simulink model "SF016A_VehSpdLimr"  (R2013b)
settings: Solver=FixedStepDiscrete  StartTime=0.0  StopTime=15  FixedStep=.002  RelTol=1e-3
values from neighbouring files (symbols this model uses):
  VehSpdLimrMaxAssiY = DataDict.Calibration    [SF016A_VehSpdLimr_DataDict.m]
  VehSpdLimrPosMaxOffs1 = DataDict.Calibration    [SF016A_VehSpdLimr_DataDict.m]
  VehSpdLimrPosMaxOffs2 = DataDict.Calibration    [SF016A_VehSpdLimr_DataDict.m]
libraries: FloatToFixd x4, NxtrAbslt x3, simulink x1, FixdToFloat x1, NxtrLim x1, LnrIntrpnDyn x1, LnrIntrpn x1
settings Model: CovHTMLOptions=-aTS=1 -bRG=1 -bTC=1 -hTR=0 -nFC=0 -scm=1 -bcm=1 -xEv=0  Creator=Praveen/Muragesh (KPIT)  LastModifiedBy=BZHF94
settings DataIOCC: SignalLoggingSaveFormat=ModelDataLogs  SaveOutput=off  SignalLogging=off  DSMLogging=off  SaveTime=off
settings OptimizationCC: ExpressionDepthLimit=2147483647
settings DebuggingCC: SolverPrmCheckMsg=none  ParameterPrecisionLossMsg=none  FcnCallInpInsideContextMsg=UseLocalSettings  StateNameClashWarn=warning
settings GRTTargetCC: CombineOutputUpdateFcns=off  GRTInterface=on

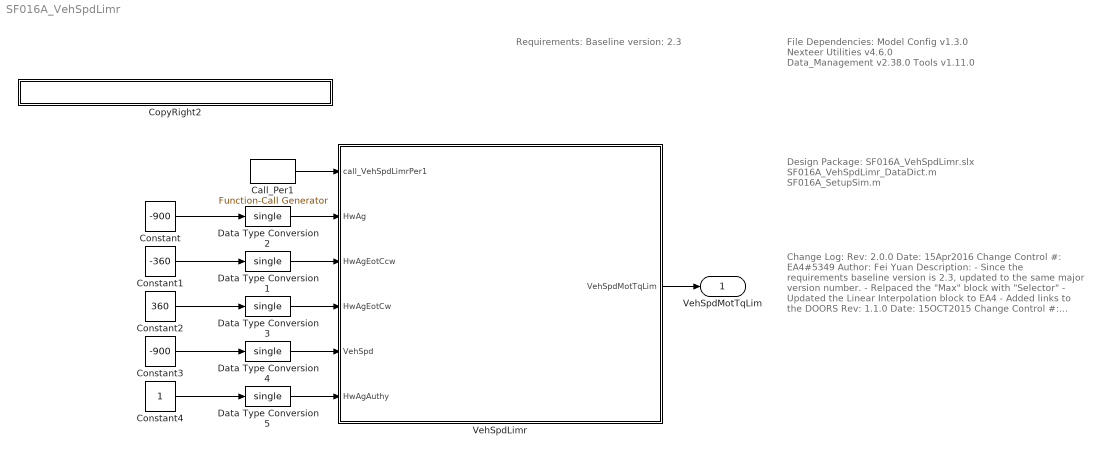
== system SF016A_VehSpdLimr ==
  note: File Dependencies:
      |
      | Model Config v1.3.0
      | Nexteer Utilities v4.6.0
      | Data_Management v2.38.0
      | Tools v1.11.0
  note: Requirements: Baseline version: 2.3
  note: Change Log:
      |
      | Rev: 2.0.0
      | Date: 15Apr2016
      | Change Control #: EA4#5349
      | Author: Fei Yuan
      | Description:
      | - Since the requirements baseline version
      |   is 2.3, updated to the same major version
      |   number.
      | - Relpaced the "Max" block with "Selector"
      | - Updated the Linear Interpolation block to
      |   EA4
      | - Added links to the DOORS
      |
      | Rev: 1.1.0
      | Date: 15OCT2015
      | Change Control #: EA4#1862
      | DRW: Praveen/Muragesh (KPIT)
      | Description:
      | Updated as per anomaly CR EA4#1276
      |
      |
      | Rev: 1.0.0
      | Date: 05AUG2015
      | Change Control #: EA4#513
      | DRW: Wheatley
      | Description:
      | Initial EA4 Release
      |  based on version EA3 v2.0
      |  this is a level 0 model
  note: Design Package:
      | SF016A_VehSpdLimr.slx
      | SF016A_VehSpdLimr_DataDict.m
      | SF016A_SetupSim.m
  Call_Per1 : simulink/Ports & Subsystems/Function-Call Generator  RequirementInfo="{'linktype_rmi_doors' '0000a52f (/E-STEER Core/SubSystem Specifications/Application Functions/SF016A Vehicle Speed Limiting)' '#SF016A_67' 'true' 'REQ:  SF016A_67' '' } %GIDa_4658042f_68a9_4f55_bcbd_8e644fae8943"  sample_time=0.002  numberOfIterations=1
  Constant : Constant  Value=-900
  Constant1 : Constant  Value=-360
  Constant2 : Constant  Value=360
  Constant3 : Constant  Value=-900
  Constant4 : Constant
  CopyRight2 : Subsystem  Description=|  mask(Copyright Information){none=on}
      | Copyright info block.                                               
      |                                                                     
      | Place copyright information at the top of every subsystem in design.
      mask prompts: none "No parameters"
      mask help: Place copyright information at the top of every subsystem in design.
      mask Display:
      | NxtrConf = 'Nexteer Confidential';
      | 
      | sys = bdroot; %handle for the current model ("system")
      | first = get_param(sys,'Created');
      | first = first(end-3:end);  %year is last four digits
      | 
      | last = get_param(sys,'LastModifiedDate');
      | if isempty(last)
      |     last = datestr(now,'yyyy');
      | else
      |     last = last(end-3:end);
      | end
      | 
      | if strcmp(first,last)
      |     fprintf('%s -- Copyright %s Nexteer',NxtrConf,first)
      | else
      |     fprintf('%s -- %s%s- %s Nexteer',NxtrConf,char(169),first,last)
      | end
  Data Type Conversion{1..5} (5 alike) : DataTypeConversion  OutDataTypeStr=single
  VehSpdLimr : Subsystem
  VehSpdMotTqLim : Outport  RequirementInfo={} %GIDa_da28f505_4b6b_4750_bcec_084d0a7cec68
  wires:
  VehSpdLimr/1(VehSpdMotTqLim) -> VehSpdMotTqLim/1
  Call_Per1/1 -> VehSpdLimr/1(call_VehSpdLimrPer1)
  Constant/1 -> Data Type Conversion2/1
  Constant1/1 -> Data Type Conversion1/1
  Constant2/1 -> Data Type Conversion3/1
  Data Type Conversion1/1 -> VehSpdLimr/3(HwAgEotCcw)
  Data Type Conversion3/1 -> VehSpdLimr/4(HwAgEotCw)
  Data Type Conversion2/1 -> VehSpdLimr/2(HwAg)
  Constant3/1 -> Data Type Conversion4/1
  Constant4/1 -> Data Type Conversion5/1
  Data Type Conversion5/1 -> VehSpdLimr/6(HwAgAuthy)
  Data Type Conversion4/1 -> VehSpdLimr/5(VehSpd)

== system SF016A_VehSpdLimr/CopyRight2 ==

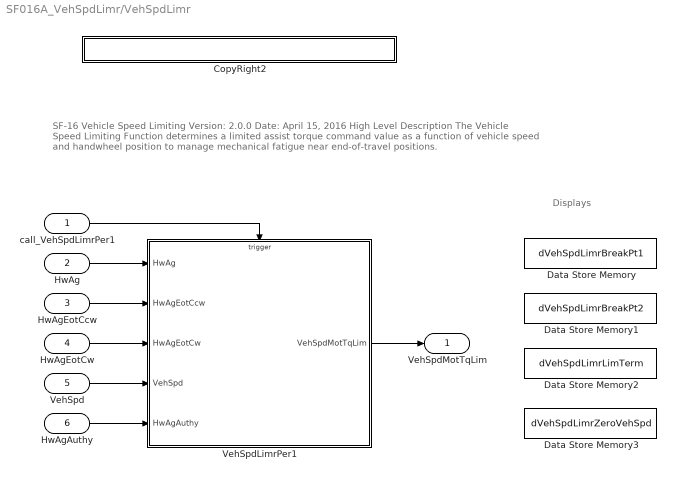
== system SF016A_VehSpdLimr/VehSpdLimr ==
  note: Displays
  note: SF-16  Vehicle Speed Limiting
      |          Version:  2.0.0                      Date:  April 15, 2016
      |
      |  High Level Description
      |      The Vehicle Speed Limiting Function determines a limited assist torque command value as a function of vehicle
      |      speed and handwheel position to manage mechanical fatigue near end-of-travel positions.
  call_VehSpdLimrPer1 : Inport
  HwAg : Inport  RequirementInfo="{'linktype_rmi_doors' '0000a52f (/E-STEER Core/SubSystem Specifications/Application Functions/SF016A Vehicle Speed Limiting)' '#SF016A_9' 'true' 'REQ:  SF016A_9' '' } %GIDa_20547f83_a8e8_4141_b0f2_e12d69f35c0f"  Port=2
  HwAgEotCcw : Inport  RequirementInfo="{'linktype_rmi_doors' '0000a52f (/E-STEER Core/SubSystem Specifications/Application Functions/SF016A Vehicle Speed Limiting)' '#SF016A_33' 'true' 'REQ:  SF016A_33' '' } %GIDa_3ac37e8a_9dbe_40a7_8cf1_05a3310f1eab"  Port=3
  HwAgEotCw : Inport  RequirementInfo="{'linktype_rmi_doors' '0000a52f (/E-STEER Core/SubSystem Specifications/Application Functions/SF016A Vehicle Speed Limiting)' '#SF016A_34' 'true' 'REQ:  SF016A_34' '' } %GIDa_e8ff42f4_7b63_425a_824a_61ddee63e2cb"  Port=4
  VehSpd : Inport  RequirementInfo="{'linktype_rmi_doors' '0000a52f (/E-STEER Core/SubSystem Specifications/Application Functions/SF016A Vehicle Speed Limiting)' '#SF016A_32' 'true' 'REQ:  SF016A_32' '' } %GIDa_d2851bec_d3f7_4000_a703_08ebed04af28"  Port=5
  HwAgAuthy : Inport  RequirementInfo="{'linktype_rmi_doors' '0000a52f (/E-STEER Core/SubSystem Specifications/Application Functions/SF016A Vehicle Speed Limiting)' '#SF016A_35' 'true' 'REQ:  SF016A_35' '' } %GIDa_755c219f_160e_44a1_8e53_1c7262d57e16"  Port=6
  CopyRight2 : Subsystem  Description=|  mask(Copyright Information){none=on}
      | Copyright info block.                                               
      |                                                                     
      | Place copyright information at the top of every subsystem in design.
      mask prompts: none "No parameters"
      mask help: Place copyright information at the top of every subsystem in design.
      mask Display:
      | NxtrConf = 'Nexteer Confidential';
      | 
      | sys = bdroot; %handle for the current model ("system")
      | first = get_param(sys,'Created');
      | first = first(end-3:end);  %year is last four digits
      | 
      | last = get_param(sys,'LastModifiedDate');
      | if isempty(last)
      |     last = datestr(now,'yyyy');
      | else
      |     last = last(end-3:end);
      | end
      | 
      | if strcmp(first,last)
      |     fprintf('%s -- Copyright %s Nexteer',NxtrConf,first)
      | else
      |     fprintf('%s -- %s%s- %s Nexteer',NxtrConf,char(169),first,last)
      | end
  Data Store Memory : DataStoreMemory  DataStoreName=dVehSpdLimrBreakPt1  ReadBeforeWriteMsg=warning  WriteAfterWriteMsg=warning  WriteAfterReadMsg=warning  StateMustResolveToSignalObject=on
  Data Store Memory1 : DataStoreMemory  DataStoreName=dVehSpdLimrBreakPt2  ReadBeforeWriteMsg=warning  WriteAfterWriteMsg=warning  WriteAfterReadMsg=warning  StateMustResolveToSignalObject=on
  Data Store Memory2 : DataStoreMemory  DataStoreName=dVehSpdLimrLimTerm  ReadBeforeWriteMsg=warning  WriteAfterWriteMsg=warning  WriteAfterReadMsg=warning  StateMustResolveToSignalObject=on
  Data Store Memory3 : DataStoreMemory  DataStoreName=dVehSpdLimrZeroVehSpd  ReadBeforeWriteMsg=warning  WriteAfterWriteMsg=warning  WriteAfterReadMsg=warning  StateMustResolveToSignalObject=on
  VehSpdLimrPer1 : Subsystem  RequirementInfo={} %GIDa_a7b0248b_b47a_44ce_9f08_25597632b35e
  VehSpdMotTqLim : Outport  RequirementInfo="{'linktype_rmi_doors' '0000a52f (/E-STEER Core/SubSystem Specifications/Application Functions/SF016A Vehicle Speed Limiting)' '#SF016A_71' 'true' 'REQ:  SF016A_71' '' } %GIDa_d0f1a28c_c8c7_42db_82c7_049fb0679538"
  wires:
  VehSpdLimrPer1/1(VehSpdMotTqLim) -> VehSpdMotTqLim/1
  HwAg/1 -> VehSpdLimrPer1/1(HwAg)
  HwAgEotCcw/1 -> VehSpdLimrPer1/2(HwAgEotCcw)
  HwAgEotCw/1 -> VehSpdLimrPer1/3(HwAgEotCw)
  call_VehSpdLimrPer1/1 -> VehSpdLimrPer1/Trigger
  VehSpd/1 -> VehSpdLimrPer1/4(VehSpd)
  HwAgAuthy/1 -> VehSpdLimrPer1/5(HwAgAuthy)

== system SF016A_VehSpdLimr/VehSpdLimr/CopyRight2 ==

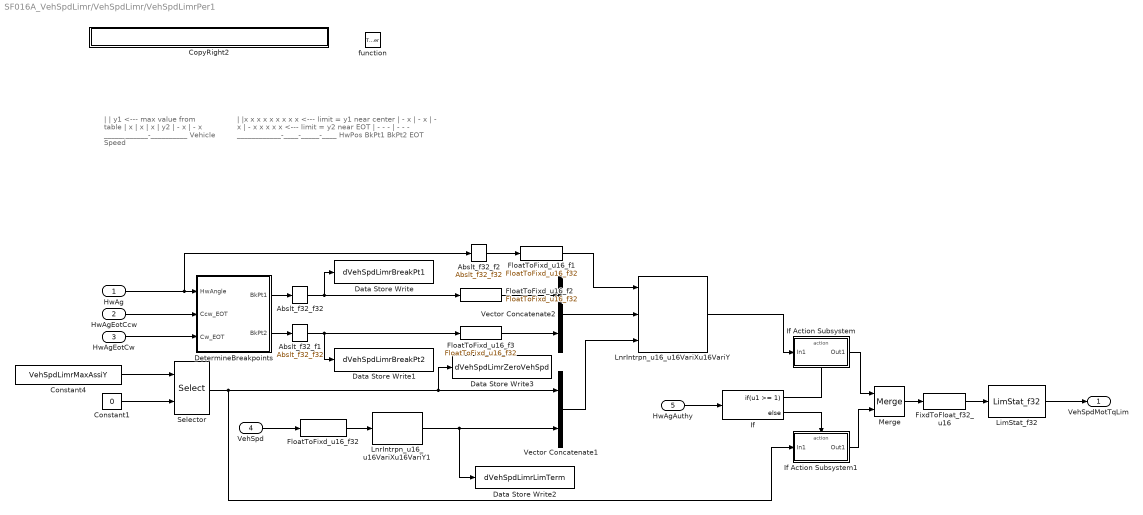
== system SF016A_VehSpdLimr/VehSpdLimr/VehSpdLimrPer1 ==
  note: |
      | | y1  <--- max value from table
      | |       x
      | |            x
      | |                 x
      | |                      y2
      | |                       -    x
      | |                       -         x
      | ____________-__________
      |               Vehicle Speed
  note: |
      | |x x x x x x x x x   <--- limit = y1 near center
      | |                       - x
      | |                       -   x
      | |                       -     x
      | |                       -        x x x x x   <--- limit = y2 near EOT
      | |                       -        -          -
      | |                       -        -          -
      | ____________-____-_____-____
      |  HwPos        BkPt1  BkPt2  EOT
  HwAg : Inport
  HwAgEotCcw : Inport  Port=2
  HwAgEotCw : Inport  Port=3
  VehSpd : Inport  Port=4
  HwAgAuthy : Inport  Port=5
  function : TriggerPort  TriggerType=function-call  PortDimensions=1
  Abslt_f32_f1 : NxtrAbslt/Abslt_f32_f32  RequirementInfo="{'linktype_rmi_doors' '0000a52f (/E-STEER Core/SubSystem Specifications/Application Functions/SF016A Vehicle Speed Limiting)' '#SF016A_56' 'true' 'REQ:  SF016A_56' '' ; 'linktype_rmi_doors' '0000a52f (/E-STEER Core/SubSystem Specifications/Application Functions/SF016A Vehicle Speed Limiting)' '#SF016A_54' 'true' 'REQ:  SF016A_54' '' } %GIDa_43263355_4d1a_4eb1_9e62_e416dfefd7d2"  SFunctionSpec=single y1 = Abslt_f32_f32(single u1)
      settings: AttributesFormatString=%<Name>
  Abslt_f32_f2 : NxtrAbslt/Abslt_f32_f32  RequirementInfo="{'linktype_rmi_doors' '0000a52f (/E-STEER Core/SubSystem Specifications/Application Functions/SF016A Vehicle Speed Limiting)' '#SF016A_56' 'true' 'REQ:  SF016A_56' '' } %GIDa_8eb8f50f_4865_40e8_a219_777cf0fc9352"  SFunctionSpec=single y1 = Abslt_f32_f32(single u1)
      settings: AttributesFormatString=%<Name>
  Abslt_f32_f32 : NxtrAbslt/Abslt_f32_f32  RequirementInfo="{'linktype_rmi_doors' '0000a52f (/E-STEER Core/SubSystem Specifications/Application Functions/SF016A Vehicle Speed Limiting)' '#SF016A_56' 'true' 'REQ:  SF016A_56' '' ; 'linktype_rmi_doors' '0000a52f (/E-STEER Core/SubSystem Specifications/Application Functions/SF016A Vehicle Speed Limiting)' '#SF016A_54' 'true' 'REQ:  SF016A_54' '' } %GIDa_6957cd74_7bb0_4d12_b411_ae19857dee05"  SFunctionSpec=single y1 = Abslt_f32_f32(single u1)
      settings: AttributesFormatString=%<Name>
  Constant1 : Constant  RequirementInfo={} %GIDa_2f2f3ffa_28ad_4d70_8ca4_c76dd9d21516  Value=0
  Constant4 : Constant  RequirementInfo="{'linktype_rmi_doors' '0000a52f (/E-STEER Core/SubSystem Specifications/Application Functions/SF016A Vehicle Speed Limiting)' '#SF016A_74' 'true' 'REQ:  SF016A_74' '' } %GIDa_3322659a_1957_4894_a58a_a65a58fad10f"  Value=VehSpdLimrMaxAssiY
  CopyRight2 : Subsystem  Description=|  mask(Copyright Information){none=on}
      | Copyright info block.                                               
      |                                                                     
      | Place copyright information at the top of every subsystem in design.
      mask prompts: none "No parameters"
      mask help: Place copyright information at the top of every subsystem in design.
      mask Display:
      | NxtrConf = 'Nexteer Confidential';
      | 
      | sys = bdroot; %handle for the current model ("system")
      | first = get_param(sys,'Created');
      | first = first(end-3:end);  %year is last four digits
      | 
      | last = get_param(sys,'LastModifiedDate');
      | if isempty(last)
      |     last = datestr(now,'yyyy');
      | else
      |     last = last(end-3:end);
      | end
      | 
      | if strcmp(first,last)
      |     fprintf('%s -- Copyright %s Nexteer',NxtrConf,first)
      | else
      |     fprintf('%s -- %s%s- %s Nexteer',NxtrConf,char(169),first,last)
      | end
  Data Store Write : DataStoreWrite  DataStoreName=dVehSpdLimrBreakPt1
  Data Store Write1 : DataStoreWrite  DataStoreName=dVehSpdLimrBreakPt2
  Data Store Write2 : DataStoreWrite  DataStoreName=dVehSpdLimrLimTerm
  Data Store Write3 : DataStoreWrite  DataStoreName=dVehSpdLimrZeroVehSpd
  DetermineBreakpoints : Subsystem  RequirementInfo="{'linktype_rmi_doors' '0000a52f (/E-STEER Core/SubSystem Specifications/Application Functions/SF016A Vehicle Speed Limiting)' '#SF016A_54' 'true' 'REQ:  SF016A_54' '' ; 'linktype_rmi_doors' '0000a52f (/E-STEER Core/SubSystem Specifications/Application Functions/SF016A Vehicle Speed Limiting)' '#SF016A_56' 'true' 'REQ:  SF016A_56' '' } %GIDa_640bd7c0_9db0_469b_8783_b292ad617612"
  FixdToFloat_f32_u16 : FixdToFloat/FixdToFloat_f32_u16  Param1=11
  FloatToFixd_u16_f1 : FloatToFixd/FloatToFixd_u16_f32  Param1=5
  FloatToFixd_u16_f2 : FloatToFixd/FloatToFixd_u16_f32  Param1=5
  FloatToFixd_u16_f3 : FloatToFixd/FloatToFixd_u16_f32  Param1=5
  FloatToFixd_u16_f32 : FloatToFixd/FloatToFixd_u16_f32  Param1=7
  If : If  RequirementInfo="{'linktype_rmi_doors' '0000a52f (/E-STEER Core/SubSystem Specifications/Application Functions/SF016A Vehicle Speed Limiting)' '#SF016A_75' 'true' 'REQ:  SF016A_75' '' ; 'linktype_rmi_doors' '0000a52f (/E-STEER Core/SubSystem Specifications/Application Functions/SF016A Vehicle Speed Limiting)' '#SF016A_54' 'true' 'REQ:  SF016A_54' '' ; 'linktype_rmi_doors' '0000a52f (/E-STEER Core/SubSystem Specifications/Application Functions/SF016A Vehicle Speed Limiting)' '#SF016A_58' 'true' 'REQ:  SF016A_58' '' ; 'linktype_rmi_doors' '0000a52f (/E-STEER Core/SubSystem Specifications/Application Functions/SF016A Vehicle Speed Limiting)' '#SF016A_59' 'true' 'REQ:  SF016A_59' '' } %GIDa_5033a59a_14fc_4531_96fc_5b75a1e94d2f"  IfExpression=u1 >= 1
  If Action Subsystem : Subsystem  RequirementInfo="{'linktype_rmi_doors' '0000a52f (/E-STEER Core/SubSystem Specifications/Application Functions/SF016A Vehicle Speed Limiting)' '#SF016A_54' 'true' 'REQ:  SF016A_54' '' ; 'linktype_rmi_doors' '0000a52f (/E-STEER Core/SubSystem Specifications/Application Functions/SF016A Vehicle Speed Limiting)' '#SF016A_58' 'true' 'REQ:  SF016A_58' '' ; 'linktype_rmi_doors' '0000a52f (/E-STEER Core/SubSystem Specifications/Application Functions/SF016A Vehicle Speed Limiting)' '#SF016A_59' 'true' 'REQ:  SF016A_59' '' } %GIDa_86a6a176_9baa_4b24_9f35_1d44feccd65f"  TreatAsAtomicUnit=on
  If Action Subsystem1 : Subsystem  RequirementInfo="{'linktype_rmi_doors' '0000a52f (/E-STEER Core/SubSystem Specifications/Application Functions/SF016A Vehicle Speed Limiting)' '#SF016A_75' 'true' 'REQ:  SF016A_75' '' ; 'linktype_rmi_doors' '0000a52f (/E-STEER Core/SubSystem Specifications/Application Functions/SF016A Vehicle Speed Limiting)' '#SF016A_58' 'true' 'REQ:  SF016A_58' '' ; 'linktype_rmi_doors' '0000a52f (/E-STEER Core/SubSystem Specifications/Application Functions/SF016A Vehicle Speed Limiting)' '#SF016A_59' 'true' 'REQ:  SF016A_59' '' } %GIDa_13070b2b_abb9_4f1f_8896_3ac05b76473f"  TreatAsAtomicUnit=on
  LimStat_f32 : NxtrLim/LimStat_f32  RequirementInfo="{'linktype_rmi_doors' '0000a52f (/E-STEER Core/SubSystem Specifications/Application Functions/SF016A Vehicle Speed Limiting)' '#SF016A_66' 'true' 'REQ:  SF016A_66' '' } %GIDa_b7f64418_05a1_4509_9d3e_29ff1aafe1ab"  LoLim=SYSGLBPRM_MOTTQCMDLOLIM_MOTNWTMTR_F32  HiLim=SYSGLBPRM_MOTTQCMDHILIM_MOTNWTMTR_F32
      settings: AttributesFormatString=|
      | Low Limit: %<LoLim>
      | High Limit:%<HiLim>
  LnrIntrpn_u16_u16VariXu16VariY : LnrIntrpnDyn/LnrIntrpn_u16_u16VariXu16VariY  RequirementInfo="{'linktype_rmi_doors' '0000a52f (/E-STEER Core/SubSystem Specifications/Application Functions/SF016A Vehicle Speed Limiting)' '#SF016A_54' 'true' 'REQ:  SF016A_54' '' ; 'linktype_rmi_doors' '0000a52f (/E-STEER Core/SubSystem Specifications/Application Functions/SF016A Vehicle Speed Limiting)' '#SF016A_56' 'true' 'REQ:  SF016A_56' '' ; 'linktype_rmi_doors' '0000a52f (/E-STEER Core/SubSystem Specifications/Application Functions/SF016A Vehicle Speed Limiting)' '#SF016A_58' 'true' 'REQ:  SF016A_58' '' ; 'linktype_rmi_doors' '0000a52f (/E-STEER Core/SubSystem Specifications/Application Functions/SF016A Vehicle Speed Limiting)' '#SF016A_59' 'true' 'REQ:  SF016A_59' '' } %GIDa_2a3c4297_300c_4538_93a7_e8369b10a31f"
      settings: AttributesFormatString=Lnr ( u16VariX , u16VariY )
  LnrIntrpn_u16_u16VariXu16VariY1 : LnrIntrpn/LnrIntrpn_u16_u16VariXu16VariY  RequirementInfo="{'linktype_rmi_doors' '0000a52f (/E-STEER Core/SubSystem Specifications/Application Functions/SF016A Vehicle Speed Limiting)' '#SF016A_58' 'true' 'REQ:  SF016A_58' '' ; 'linktype_rmi_doors' '0000a52f (/E-STEER Core/SubSystem Specifications/Application Functions/SF016A Vehicle Speed Limiting)' '#SF016A_59' 'true' 'REQ:  SF016A_59' '' ; 'linktype_rmi_doors' '0000a52f (/E-STEER Core/SubSystem Specifications/Application Functions/SF016A Vehicle Speed Limiting)' '#SF016A_63' 'true' 'REQ:  SF016A_63' '' } %GIDa_7e84c74c_bad8_4c0d_9f88_70828bbee0f2"  XTbl=VehSpdLimrMaxAssiX  YTbl=VehSpdLimrMaxAssiY
      settings: AttributesFormatString=Lnr ( u16VariX , u16VariY )
  Merge : Merge  RequirementInfo="{'linktype_rmi_doors' '0000a52f (/E-STEER Core/SubSystem Specifications/Application Functions/SF016A Vehicle Speed Limiting)' '#SF016A_75' 'true' 'REQ:  SF016A_75' '' ; 'linktype_rmi_doors' '0000a52f (/E-STEER Core/SubSystem Specifications/Application Functions/SF016A Vehicle Speed Limiting)' '#SF016A_54' 'true' 'REQ:  SF016A_54' '' ; 'linktype_rmi_doors' '0000a52f (/E-STEER Core/SubSystem Specifications/Application Functions/SF016A Vehicle Speed Limiting)' '#SF016A_58' 'true' 'REQ:  SF016A_58' '' ; 'linktype_rmi_doors' '0000a52f (/E-STEER Core/SubSystem Specifications/Application Functions/SF016A Vehicle Speed Limiting)' '#SF016A_59' 'true' 'REQ:  SF016A_59' '' } %GIDa_04d40666_89e5_49bf_be68_7e9bf64bae41"
  Selector : Selector  RequirementInfo="{'linktype_rmi_doors' '0000a52f (/E-STEER Core/SubSystem Specifications/Application Functions/SF016A Vehicle Speed Limiting)' '#SF016A_75' 'true' 'REQ:  SF016A_75' '' } %GIDa_ed021c59_1b39_418e_9ab3_afd0e64960ef"  IndexMode=Zero-based  InputPortWidth=5  IndexOptions=Index vector (port)  Indices=[1 3]  OutputSizes=1
  Vector Concatenate1 : Concatenate  RequirementInfo="{'linktype_rmi_doors' '0000a52f (/E-STEER Core/SubSystem Specifications/Application Functions/SF016A Vehicle Speed Limiting)' '#SF016A_54' 'true' 'REQ:  SF016A_54' '' ; 'linktype_rmi_doors' '0000a52f (/E-STEER Core/SubSystem Specifications/Application Functions/SF016A Vehicle Speed Limiting)' '#SF016A_56' 'true' 'REQ:  SF016A_56' '' ; 'linktype_rmi_doors' '0000a52f (/E-STEER Core/SubSystem Specifications/Application Functions/SF016A Vehicle Speed Limiting)' '#SF016A_58' 'true' 'REQ:  SF016A_58' '' ; 'linktype_rmi_doors' '0000a52f (/E-STEER Core/SubSystem Specifications/Application Functions/SF016A Vehicle Speed Limiting)' '#SF016A_59' 'true' 'REQ:  SF016A_59' '' } %GIDa_aa604e0a_c245_4d50_bf5a_9e569c9abc5e"
  Vector Concatenate2 : Concatenate  RequirementInfo="{'linktype_rmi_doors' '0000a52f (/E-STEER Core/SubSystem Specifications/Application Functions/SF016A Vehicle Speed Limiting)' '#SF016A_54' 'true' 'REQ:  SF016A_54' '' ; 'linktype_rmi_doors' '0000a52f (/E-STEER Core/SubSystem Specifications/Application Functions/SF016A Vehicle Speed Limiting)' '#SF016A_56' 'true' 'REQ:  SF016A_56' '' ; 'linktype_rmi_doors' '0000a52f (/E-STEER Core/SubSystem Specifications/Application Functions/SF016A Vehicle Speed Limiting)' '#SF016A_58' 'true' 'REQ:  SF016A_58' '' ; 'linktype_rmi_doors' '0000a52f (/E-STEER Core/SubSystem Specifications/Application Functions/SF016A Vehicle Speed Limiting)' '#SF016A_59' 'true' 'REQ:  SF016A_59' '' } %GIDa_62854488_0536_41b3_903d_0888355aa9ab"
  VehSpdMotTqLim : Outport
  wires:
  DetermineBreakpoints/1(BkPt1) -> Abslt_f32_f32/1
  DetermineBreakpoints/2(BkPt2) -> Abslt_f32_f1/1
  HwAgAuthy/1 -> If/1
  HwAgEotCcw/1 -> DetermineBreakpoints/2(Ccw_EOT)
  HwAgEotCw/1 -> DetermineBreakpoints/3(Cw_EOT)
  Abslt_f32_f2/1 -> FloatToFixd_u16_f1/1
  HwAg/1 -> Abslt_f32_f2/1, DetermineBreakpoints/1(HwAngle)
  If/1 -> If Action Subsystem/Action
  If/2 -> If Action Subsystem1/Action
  If Action Subsystem/1(Out1) -> Merge/1
  If Action Subsystem1/1(Out1) -> Merge/2
  Merge/1 -> FixdToFloat_f32_u16/1
  LnrIntrpn_u16_u16VariXu16VariY/1 -> If Action Subsystem/1(In1)
  LimStat_f32/1 -> VehSpdMotTqLim/1
  FixdToFloat_f32_u16/1 -> LimStat_f32/1
  Vector Concatenate2/1 -> LnrIntrpn_u16_u16VariXu16VariY/2
  FloatToFixd_u16_f1/1 -> LnrIntrpn_u16_u16VariXu16VariY/1
  FloatToFixd_u16_f2/1 -> Vector Concatenate2/1
  FloatToFixd_u16_f3/1 -> Vector Concatenate2/2
  VehSpd/1 -> FloatToFixd_u16_f32/1
  FloatToFixd_u16_f32/1 -> LnrIntrpn_u16_u16VariXu16VariY1/1
  LnrIntrpn_u16_u16VariXu16VariY1/1 -> Data Store Write2/1, Vector Concatenate1/2
  Abslt_f32_f32/1 -> Data Store Write/1, FloatToFixd_u16_f2/1
  Abslt_f32_f1/1 -> Data Store Write1/1, FloatToFixd_u16_f3/1
  Selector/1 -> If Action Subsystem1/1(In1), Vector Concatenate1/1, Data Store Write3/1
  Vector Concatenate1/1 -> LnrIntrpn_u16_u16VariXu16VariY/3
  Constant1/1 -> Selector/2
  Constant4/1 -> Selector/1

== system SF016A_VehSpdLimr/VehSpdLimr/VehSpdLimrPer1/CopyRight2 ==

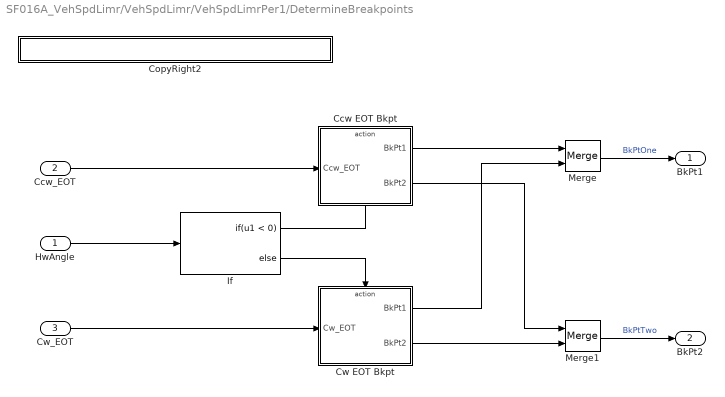
== system SF016A_VehSpdLimr/VehSpdLimr/VehSpdLimrPer1/DetermineBreakpoints ==
  HwAngle : Inport
  Ccw_EOT : Inport  Port=2
  Cw_EOT : Inport  Port=3
  Ccw EOT Bkpt : Subsystem  RequirementInfo="{'linktype_rmi_doors' '0000a52f (/E-STEER Core/SubSystem Specifications/Application Functions/SF016A Vehicle Speed Limiting)' '#SF016A_54' 'true' 'REQ:  SF016A_54' '' ; 'linktype_rmi_doors' '0000a52f (/E-STEER Core/SubSystem Specifications/Application Functions/SF016A Vehicle Speed Limiting)' '#SF016A_56' 'true' 'REQ:  SF016A_56' '' } %GIDa_e3c79417_19a6_48dc_9488_a36fc9b8a269"  TreatAsAtomicUnit=on
  CopyRight2 : Subsystem  Description=|  mask(Copyright Information){none=on}
      | Copyright info block.                                               
      |                                                                     
      | Place copyright information at the top of every subsystem in design.
      mask prompts: none "No parameters"
      mask help: Place copyright information at the top of every subsystem in design.
      mask Display:
      | NxtrConf = 'Nexteer Confidential';
      | 
      | sys = bdroot; %handle for the current model ("system")
      | first = get_param(sys,'Created');
      | first = first(end-3:end);  %year is last four digits
      | 
      | last = get_param(sys,'LastModifiedDate');
      | if isempty(last)
      |     last = datestr(now,'yyyy');
      | else
      |     last = last(end-3:end);
      | end
      | 
      | if strcmp(first,last)
      |     fprintf('%s -- Copyright %s Nexteer',NxtrConf,first)
      | else
      |     fprintf('%s -- %s%s- %s Nexteer',NxtrConf,char(169),first,last)
      | end
  Cw EOT Bkpt : Subsystem  RequirementInfo="{'linktype_rmi_doors' '0000a52f (/E-STEER Core/SubSystem Specifications/Application Functions/SF016A Vehicle Speed Limiting)' '#SF016A_54' 'true' 'REQ:  SF016A_54' '' ; 'linktype_rmi_doors' '0000a52f (/E-STEER Core/SubSystem Specifications/Application Functions/SF016A Vehicle Speed Limiting)' '#SF016A_56' 'true' 'REQ:  SF016A_56' '' } %GIDa_adf71e24_21ac_428d_a2e4_a099c634c138"  TreatAsAtomicUnit=on
  If : If  RequirementInfo="{'linktype_rmi_doors' '0000a52f (/E-STEER Core/SubSystem Specifications/Application Functions/SF016A Vehicle Speed Limiting)' '#SF016A_54' 'true' 'REQ:  SF016A_54' '' ; 'linktype_rmi_doors' '0000a52f (/E-STEER Core/SubSystem Specifications/Application Functions/SF016A Vehicle Speed Limiting)' '#SF016A_56' 'true' 'REQ:  SF016A_56' '' } %GIDa_c3b2335f_bbf3_490b_aa88_e7162cc8d21d"  IfExpression=u1 < 0
  Merge : Merge  RequirementInfo="{'linktype_rmi_doors' '0000a52f (/E-STEER Core/SubSystem Specifications/Application Functions/SF016A Vehicle Speed Limiting)' '#SF016A_54' 'true' 'REQ:  SF016A_54' '' ; 'linktype_rmi_doors' '0000a52f (/E-STEER Core/SubSystem Specifications/Application Functions/SF016A Vehicle Speed Limiting)' '#SF016A_56' 'true' 'REQ:  SF016A_56' '' } %GIDa_04a606ba_b5f0_43c7_bb3d_819425f6e791"
  Merge1 : Merge  RequirementInfo="{'linktype_rmi_doors' '0000a52f (/E-STEER Core/SubSystem Specifications/Application Functions/SF016A Vehicle Speed Limiting)' '#SF016A_54' 'true' 'REQ:  SF016A_54' '' ; 'linktype_rmi_doors' '0000a52f (/E-STEER Core/SubSystem Specifications/Application Functions/SF016A Vehicle Speed Limiting)' '#SF016A_56' 'true' 'REQ:  SF016A_56' '' } %GIDa_5b2318de_e3dc_4ba1_8390_700fb8f2154c"
  BkPt1 : Outport
  BkPt2 : Outport  Port=2
  wires:
  Ccw_EOT/1 -> Ccw EOT Bkpt/1(Ccw_EOT)
  Cw_EOT/1 -> Cw EOT Bkpt/1(Cw_EOT)
  If/1 -> Ccw EOT Bkpt/Action
  If/2 -> Cw EOT Bkpt/Action
  Ccw EOT Bkpt/1(BkPt1) -> Merge/1
  Cw EOT Bkpt/1(BkPt1) -> Merge/2
  Ccw EOT Bkpt/2(BkPt2) -> Merge1/1
  Cw EOT Bkpt/2(BkPt2) -> Merge1/2
  HwAngle/1 -> If/1
  Merge/1 -> BkPt1/1  "BkPtOne"
  Merge1/1 -> BkPt2/1  "BkPtTwo"

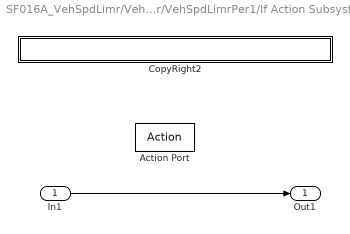
== system SF016A_VehSpdLimr/VehSpdLimr/VehSpdLimrPer1/If Action Subsystem ==
  In1 : Inport
  Action Port : ActionPort  ActionType=then
  CopyRight2 : Subsystem  Description=|  mask(Copyright Information){none=on}
      | Copyright info block.                                               
      |                                                                     
      | Place copyright information at the top of every subsystem in design.
      mask prompts: none "No parameters"
      mask help: Place copyright information at the top of every subsystem in design.
      mask Display:
      | NxtrConf = 'Nexteer Confidential';
      | 
      | sys = bdroot; %handle for the current model ("system")
      | first = get_param(sys,'Created');
      | first = first(end-3:end);  %year is last four digits
      | 
      | last = get_param(sys,'LastModifiedDate');
      | if isempty(last)
      |     last = datestr(now,'yyyy');
      | else
      |     last = last(end-3:end);
      | end
      | 
      | if strcmp(first,last)
      |     fprintf('%s -- Copyright %s Nexteer',NxtrConf,first)
      | else
      |     fprintf('%s -- %s%s- %s Nexteer',NxtrConf,char(169),first,last)
      | end
  Out1 : Outport
  wires:
  In1/1 -> Out1/1

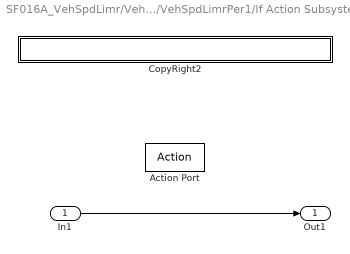
== system SF016A_VehSpdLimr/VehSpdLimr/VehSpdLimrPer1/If Action Subsystem1 ==
  In1 : Inport
  Action Port : ActionPort  ActionType=else
  CopyRight2 : Subsystem  Description=|  mask(Copyright Information){none=on}
      | Copyright info block.                                               
      |                                                                     
      | Place copyright information at the top of every subsystem in design.
      mask prompts: none "No parameters"
      mask help: Place copyright information at the top of every subsystem in design.
      mask Display:
      | NxtrConf = 'Nexteer Confidential';
      | 
      | sys = bdroot; %handle for the current model ("system")
      | first = get_param(sys,'Created');
      | first = first(end-3:end);  %year is last four digits
      | 
      | last = get_param(sys,'LastModifiedDate');
      | if isempty(last)
      |     last = datestr(now,'yyyy');
      | else
      |     last = last(end-3:end);
      | end
      | 
      | if strcmp(first,last)
      |     fprintf('%s -- Copyright %s Nexteer',NxtrConf,first)
      | else
      |     fprintf('%s -- %s%s- %s Nexteer',NxtrConf,char(169),first,last)
      | end
  Out1 : Outport
  wires:
  In1/1 -> Out1/1

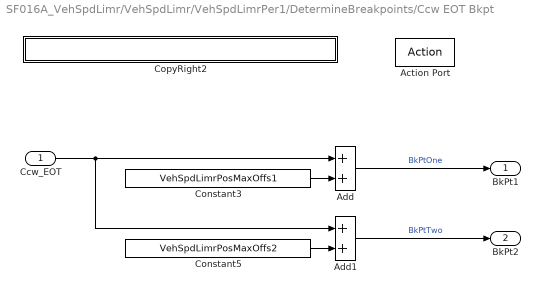
== system SF016A_VehSpdLimr/VehSpdLimr/VehSpdLimrPer1/DetermineBreakpoints/Ccw EOT Bkpt ==
  Ccw_EOT : Inport
  Action Port : ActionPort  ActionType=then
  Add : Sum  RequirementInfo="{'linktype_rmi_doors' '0000a52f (/E-STEER Core/SubSystem Specifications/Application Functions/SF016A Vehicle Speed Limiting)' '#SF016A_61' 'true' 'REQ:  SF016A_61' '' } %GIDa_b3801fec_f8e8_4979_97e6_a2343a16ea21"
  Add1 : Sum  RequirementInfo="{'linktype_rmi_doors' '0000a52f (/E-STEER Core/SubSystem Specifications/Application Functions/SF016A Vehicle Speed Limiting)' '#SF016A_62' 'true' 'REQ:  SF016A_62' '' } %GIDa_39bae563_2591_4b9f_ad28_0357182f1eb7"
  Constant3 : Constant  RequirementInfo="{'linktype_rmi_doors' '0000a52f (/E-STEER Core/SubSystem Specifications/Application Functions/SF016A Vehicle Speed Limiting)' '#SF016A_61' 'true' 'REQ:  SF016A_61' '' } %GIDa_66d15d56_bc81_42e3_bcd0_8a3b5ee1f4d3"  Value=VehSpdLimrPosMaxOffs1
  Constant5 : Constant  RequirementInfo="{'linktype_rmi_doors' '0000a52f (/E-STEER Core/SubSystem Specifications/Application Functions/SF016A Vehicle Speed Limiting)' '#SF016A_62' 'true' 'REQ:  SF016A_62' '' } %GIDa_c86c2d4f_1f1d_4609_ae27_bb0b7f5715ab"  Value=VehSpdLimrPosMaxOffs2
  CopyRight2 : Subsystem  Description=|  mask(Copyright Information){none=on}
      | Copyright info block.                                               
      |                                                                     
      | Place copyright information at the top of every subsystem in design.
      mask prompts: none "No parameters"
      mask help: Place copyright information at the top of every subsystem in design.
      mask Display:
      | NxtrConf = 'Nexteer Confidential';
      | 
      | sys = bdroot; %handle for the current model ("system")
      | first = get_param(sys,'Created');
      | first = first(end-3:end);  %year is last four digits
      | 
      | last = get_param(sys,'LastModifiedDate');
      | if isempty(last)
      |     last = datestr(now,'yyyy');
      | else
      |     last = last(end-3:end);
      | end
      | 
      | if strcmp(first,last)
      |     fprintf('%s -- Copyright %s Nexteer',NxtrConf,first)
      | else
      |     fprintf('%s -- %s%s- %s Nexteer',NxtrConf,char(169),first,last)
      | end
  BkPt1 : Outport
  BkPt2 : Outport  Port=2
  wires:
  Ccw_EOT/1 -> Add/1, Add1/1
  Constant3/1 -> Add/2
  Add/1 -> BkPt1/1  "BkPtOne"
  Constant5/1 -> Add1/2
  Add1/1 -> BkPt2/1  "BkPtTwo"

== system SF016A_VehSpdLimr/VehSpdLimr/VehSpdLimrPer1/DetermineBreakpoints/CopyRight2 ==

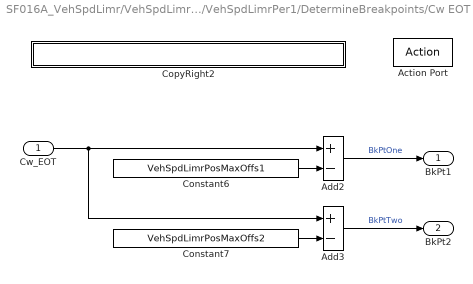
== system SF016A_VehSpdLimr/VehSpdLimr/VehSpdLimrPer1/DetermineBreakpoints/Cw EOT Bkpt ==
  Cw_EOT : Inport
  Action Port : ActionPort  ActionType=else
  Add2 : Sum  RequirementInfo="{'linktype_rmi_doors' '0000a52f (/E-STEER Core/SubSystem Specifications/Application Functions/SF016A Vehicle Speed Limiting)' '#SF016A_61' 'true' 'REQ:  SF016A_61' '' } %GIDa_8c079889_0248_4e08_800b_0d39e26c5b9e"  Inputs=+-
  Add3 : Sum  RequirementInfo="{'linktype_rmi_doors' '0000a52f (/E-STEER Core/SubSystem Specifications/Application Functions/SF016A Vehicle Speed Limiting)' '#SF016A_62' 'true' 'REQ:  SF016A_62' '' } %GIDa_5232dd6e_b17a_4e57_9522_b512f3e399d8"  Inputs=+-
  Constant6 : Constant  RequirementInfo="{'linktype_rmi_doors' '0000a52f (/E-STEER Core/SubSystem Specifications/Application Functions/SF016A Vehicle Speed Limiting)' '#SF016A_61' 'true' 'REQ:  SF016A_61' '' } %GIDa_8c3abd57_3412_4b35_b8e5_451f0f7225ed"  Value=VehSpdLimrPosMaxOffs1
  Constant7 : Constant  RequirementInfo="{'linktype_rmi_doors' '0000a52f (/E-STEER Core/SubSystem Specifications/Application Functions/SF016A Vehicle Speed Limiting)' '#SF016A_62' 'true' 'REQ:  SF016A_62' '' } %GIDa_f4fc982b_3fea_4ebf_bb74_65892309d805"  Value=VehSpdLimrPosMaxOffs2
  CopyRight2 : Subsystem  Description=|  mask(Copyright Information){none=on}
      | Copyright info block.                                               
      |                                                                     
      | Place copyright information at the top of every subsystem in design.
      mask prompts: none "No parameters"
      mask help: Place copyright information at the top of every subsystem in design.
      mask Display:
      | NxtrConf = 'Nexteer Confidential';
      | 
      | sys = bdroot; %handle for the current model ("system")
      | first = get_param(sys,'Created');
      | first = first(end-3:end);  %year is last four digits
      | 
      | last = get_param(sys,'LastModifiedDate');
      | if isempty(last)
      |     last = datestr(now,'yyyy');
      | else
      |     last = last(end-3:end);
      | end
      | 
      | if strcmp(first,last)
      |     fprintf('%s -- Copyright %s Nexteer',NxtrConf,first)
      | else
      |     fprintf('%s -- %s%s- %s Nexteer',NxtrConf,char(169),first,last)
      | end
  BkPt1 : Outport
  BkPt2 : Outport  Port=2
  wires:
  Cw_EOT/1 -> Add2/1, Add3/1
  Constant6/1 -> Add2/2
  Add2/1 -> BkPt1/1  "BkPtOne"
  Constant7/1 -> Add3/2
  Add3/1 -> BkPt2/1  "BkPtTwo"

== system SF016A_VehSpdLimr/VehSpdLimr/VehSpdLimrPer1/If Action Subsystem/CopyRight2 ==

== system SF016A_VehSpdLimr/VehSpdLimr/VehSpdLimrPer1/If Action Subsystem1/CopyRight2 ==

== system SF016A_VehSpdLimr/VehSpdLimr/VehSpdLimrPer1/DetermineBreakpoints/Ccw EOT Bkpt/CopyRight2 ==

== system SF016A_VehSpdLimr/VehSpdLimr/VehSpdLimrPer1/DetermineBreakpoints/Cw EOT Bkpt/CopyRight2 ==
